simulink model "QuadcopterModel"  (R2021b)
settings: Solver=VariableStepAuto  StartTime=0  StopTime=20  RelTol=1e-3
values from neighbouring files (symbols this model uses):
  b = 3.59 * 10^(-5)    (= 3.59e-05)    [LQR_controller.m]
  d = 2.081 * 10^(-6)    (= 2.081e-06)    [LQR_controller.m]
  g = 9.81    [LQR_controller.m]
  Ix = 0.00963    [LQR_controller.m]
  Iy = 0.00963    [LQR_controller.m]
  Iz = 0.019    [LQR_controller.m]
  Jr = 5.225 * 10^(-5)    (= 5.225e-05)    [LQR_controller.m]
  l = 0.24    [LQR_controller.m]
  m = 0.9928    [LQR_controller.m]
undefined symbols (not defined in the file or in its folder): rad, s, sigbuilder_block
libraries: slpidlib x7, simulink_extras x2, aerolibconvert2 x1
settings Model: Creator=sevba  LastModifiedBy=SEVBAN ALTAY
settings SolverCC: ZeroCrossAlgorithm=Adaptive
settings DataIOCC: SaveFormat=StructureWithTime
settings OptimizationCC: BlockReduction=off  BufferReuse=off
settings DebuggingCC: AlgebraicLoopMsg=none  IgnoredZcDiagnostic=none  UnconnectedInputMsg=none  UnconnectedOutputMsg=none  UnconnectedLineMsg=none
settings ExplorerConfigSet: SimMechanicsOpenEditorOnUpdate=off

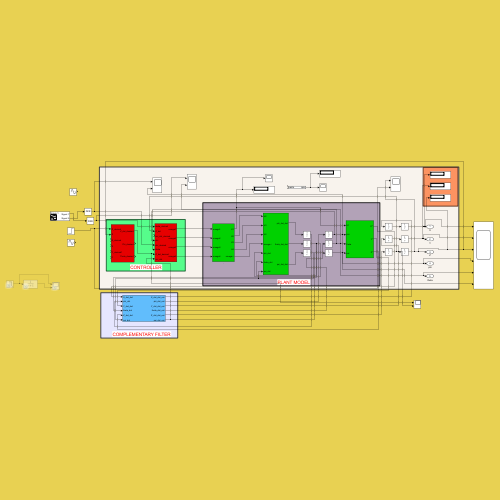
[thumbnail: Simulink's stored preview of the top-level diagram]
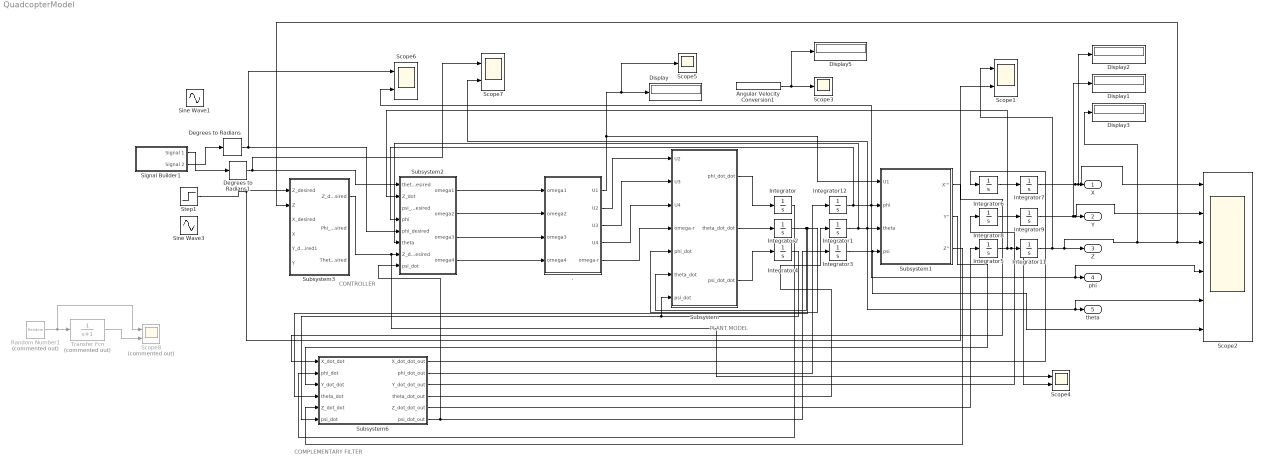
== system QuadcopterModel ==
  note: PLANT MODEL
  note: CONTROLLER
  note: COMPLEMENTARY FILTER
  . : Subsystem
  Angular Velocity Conversion1 : aerolibconvert2/Angular Velocity Conversion  IU=rad/s  OU=rpm
  Degrees to Radians : simulink_extras/Transformations/Degrees to Radians
  Degrees to Radians1 : simulink_extras/Transformations/Degrees to Radians
  Display{,1..3,5} (5 alike) : Display
  Integrator{,1..7,9,12} (10 alike) : Integrator
  Integrator11 : Integrator  UpperSaturationLimit=0  WrappedStateUpperValue=0
  Integrator8 : Integrator  UpperSaturationLimit=0
  Random Number1 : RandomNumber  Commented=on  Variance=0.0001  Seed=1  SampleTime=0.01
  Scope{1,4,6..7} (4 alike) : Scope  NumInputPorts=2
  Scope2 : Scope  NumInputPorts=6
  Scope3 : Scope
  Scope5 : Scope
  Scope8 : Scope  Commented=on  NumInputPorts=2
  Signal Builder1 : Subsystem  Tag=STV Subsys  LoadFcn=sigbuilder_block('load');  StartFcn=sigbuilder_block('start');  StopFcn=sigbuilder_block('stop');  ClipboardFcn=sigbuilder_block('clipboard');  mask(Sigbuilder block){tuvar=[0:10]}
      mask help: Simulink:masks:SigbuilderBlock_MD
      mask init:
      | if ~strcmp(get_param(bdroot(gcbh),'SimulationStatus'),'stopped') tuvar = sigbuilder_block('maskInit'); end
      settings: CopyFcn=sigbuilder_block('copy');  DeleteFcn=sigbuilder_block('delete');  ModelCloseFcn=sigbuilder_block('modelClose');  PreSaveFcn=sigbuilder_block('preSave');  PauseFcn=sigbuilder_block('pause');  ContinueFcn=sigbuilder_block('continue');  NameChangeFcn=sigbuilder_block('namechange');  OpenFcn=sigbuilder_block('open',[182.4 96.6 550.8 400.2 ]);  CloseFcn=sigbuilder_block('close');
      mask Display: plot(0, 0, 100, 100,[2, 2, 32, 32, 2], [68, 8, 8, 68, 68],[32, 2], [38, 38], [32, 19, 2],[53, 60, 44], [32, 17, 17, 2],[16, 16, 31, 31]);txt = getActiveGroup(gcbh);text(2, 100, txt,'verticalAlignment', 'top');
  Sine Wave1 : Sin  SampleTime=0
  Sine Wave3 : Sin  SampleTime=0
  Step1 : Step  SampleTime=0
  Subsystem : Subsystem
  Subsystem1 : Subsystem
  Subsystem2 : Subsystem
  Subsystem3 : Subsystem
  Subsystem6 : Subsystem
  Transfer Fcn : TransferFcn  Commented=on  Denominator=[1 1]
  X : Outport
  "Y " : Outport  Port=2
  Z : Outport  Port=3
  phi : Outport  Port=4
  "theta " : Outport  Port=5
  wires:
  Integrator5/1 -> Scope4/2, Integrator11/1, Subsystem2/2(Z_dot)
  Integrator8/1 -> Integrator9/1
  ./3(U3) -> Subsystem/2(U3)
  ./1(U1) -> Scope5/1, Display/1, Subsystem1/1(U1)
  Integrator3/1 -> Subsystem1/4(psi), Scope2/6
  Subsystem/3(psi_dot_dot) -> Integrator4/1
  Subsystem/2(theta_dot_dot) -> Integrator2/1
  ./2(U2) -> Subsystem/1(U2)
  Integrator2/1 -> Subsystem6/4(theta_dot), Subsystem/5(phi_dot), Subsystem/6(theta_dot)
  Integrator11/1 -> Scope1/1, Subsystem3/2(Z), Scope2/3, Display3/1, Z/1
  Integrator9/1 -> Display1/1, Scope2/2, "Y "/1
  Integrator6/1 -> Integrator7/1
  Integrator12/1 -> Subsystem2/4(phi), phi/1, Scope2/4, Subsystem1/2(phi), Scope6/2
  Subsystem/1(phi_dot_dot) -> Integrator/1
  Integrator4/1 -> Subsystem6/6(psi_dot), Subsystem/7(psi_dot)
  Integrator1/1 -> Subsystem2/6(theta), Scope2/5, "theta "/1, Scope7/2, Subsystem1/3(theta)
  ./4(U4) -> Subsystem/3(U4)
  Angular Velocity Conversion1/1 -> Display5/1, Scope3/1
  Integrator7/1 -> Scope2/1, Display2/1, X/1
  ./5(omega-r) -> Subsystem/4(omega-r)
  Subsystem2/1(omega1) -> ./1(omega1)
  Subsystem2/2(omega2) -> ./2(omega2)
  Subsystem2/3(omega3) -> ./3(omega3)
  Subsystem2/4(omega4) -> ./4(omega4)
  Step1/1 -> Scope1/2, Subsystem3/1(Z_desired)
  Subsystem3/1(Z_dot_desired) -> Scope4/1, Subsystem2/7(Z_dot_desired)
  Degrees to Radians/1 -> Subsystem2/5(phi_desired), Scope6/1
  Subsystem6/6(psi_dot_out) -> Subsystem2/8(psi_dot), Integrator3/1
  Subsystem1/1(X''') -> Subsystem6/1(X_dot_dot)
  Integrator/1 -> Subsystem6/2(phi_dot)
  Subsystem1/2(Y'') -> Subsystem6/3(Y_dot_dot)
  Subsystem6/1(X_dot_dot_out) -> Integrator6/1
  Subsystem6/2(phi_dot_out) -> Integrator12/1
  Subsystem6/3(Y_dot_dot_out) -> Integrator8/1
  Subsystem6/4(theta_dot_out) -> Integrator1/1
  Subsystem6/5(Z_dot_dot_out) -> Integrator5/1
  Subsystem1/3(Z'') -> Subsystem6/5(Z_dot_dot)
  Degrees to Radians1/1 -> Scope7/1, Subsystem2/1(theta_desired)
  Signal Builder1/2(Signal 2) -> Degrees to Radians/1
  Signal Builder1/1(Signal 1) -> Degrees to Radians1/1
  Random Number1/1 -> Scope8/1, Transfer Fcn/1
  Transfer Fcn/1 -> Scope8/2

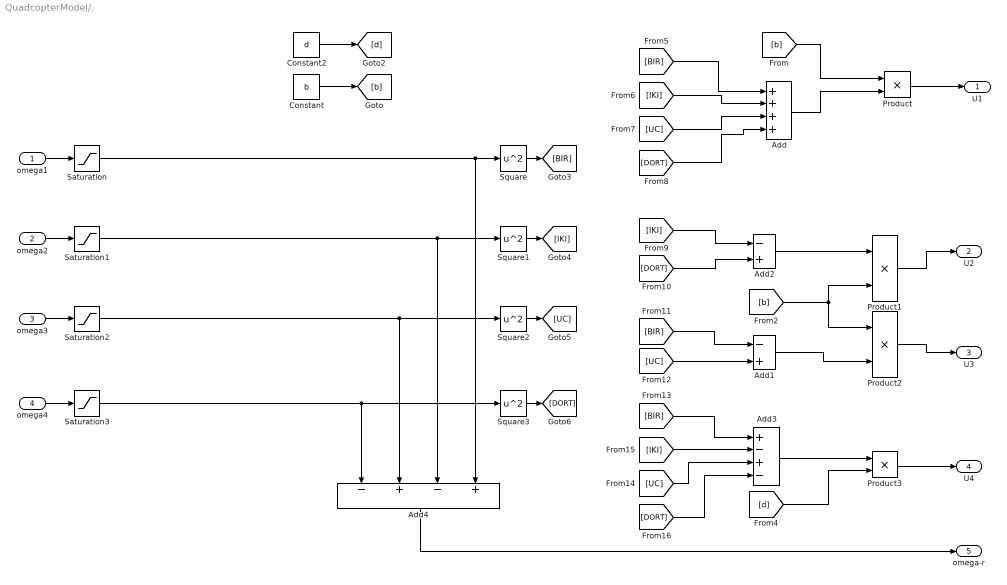
== system QuadcopterModel/. ==
  omega1 : Inport
  omega2 : Inport  Port=2
  omega3 : Inport  Port=3
  omega4 : Inport  Port=4
  Add : Sum  Inputs=++++
  Add1 : Sum  Inputs=-+
  Add2 : Sum  Inputs=-+
  Add3 : Sum  Inputs=+-+-
  Add4 : Sum  Inputs=-+-+
  Constant : Constant  Value=b
  Constant2 : Constant  Value=d
  Product{,1..3} (4 alike) : Product
  Saturation{,1..3} (4 alike) : Saturate  UpperLimit=inf  LowerLimit=0
  Square{,1..3} (4 alike) : Math  Operator=square  SaturateOnIntegerOverflow=on
  U1 : Outport
  U2 : Outport  Port=2
  U3 : Outport  Port=3
  U4 : Outport  Port=4
  omega-r : Outport  Port=5
  wires:
  Add/1 -> Product/2
  Product/1 -> U1/1
  Constant/1 -> [b]
  [b] -> Product/1
  Add2/1 -> Product1/1
  [b] -> Product1/2, Product2/1
  Add1/1 -> Product2/2
  Constant2/1 -> [d]
  Add3/1 -> Product3/1
  [d] -> Product3/2
  Product1/1 -> U2/1
  Product3/1 -> U4/1
  Product2/1 -> U3/1
  Square/1 -> [BIR]
  [BIR] -> Add/1
  Square1/1 -> [IKI]
  [IKI] -> Add/2
  Square2/1 -> [UC]
  [UC] -> Add/3
  Square3/1 -> [DORT]
  [DORT] -> Add/4
  [IKI] -> Add2/1
  [DORT] -> Add2/2
  [BIR] -> Add1/1
  [UC] -> Add1/2
  [BIR] -> Add3/1
  [UC] -> Add3/3
  [IKI] -> Add3/2
  [DORT] -> Add3/4
  Add4/1 -> omega-r/1
  omega1/1 -> Saturation/1
  omega2/1 -> Saturation1/1
  omega3/1 -> Saturation2/1
  omega4/1 -> Saturation3/1
  Saturation/1 -> Add4/4, Square/1
  Saturation1/1 -> Add4/3, Square1/1
  Saturation2/1 -> Add4/2, Square2/1
  Saturation3/1 -> Square3/1, Add4/1

== system QuadcopterModel/Signal Builder1 ==
  Demux : Demux  Tag=STV Demux  Outputs=2
      settings: DisplayOption=none
  FromWs : FromWorkspace  Tag=STV FromWs  VariableName=tuvar
      SigBuilderData=|
      | common.afterFinalStr = 'Extrapolate'
      | common.sampleTime = 0
      | dataSet.timeRange = [0 10]
      | dataSet.name = 'Group 1'
      | sbobj.Groups.Name = 'Group 1'
      | sbobj.Groups.Signals(1).Name = 'Signal 1'
      | sbobj.Groups.Signals(1).XData = [0 4 4 6 6 10]
      | sbobj.Groups.Signals(1).YData = [0 0 2.9 2.9 0 0]
      | sbobj.Groups.Signals(2).Name = 'Signal 2'
      | sbobj.Groups.Signals(2).XData = [0 4 4 6 6 10]
      | sbobj.Groups.Signals(2).YData = [0 0 -2.9 -2.9 0 0]
  Signal 1 : Outport  Tag=STV Outport
  Signal 2 : Outport  Tag=STV Outport  Port=2
  wires:
  FromWs/1 -> Demux/1
  Demux/1 -> Signal 1/1
  Demux/2 -> Signal 2/1

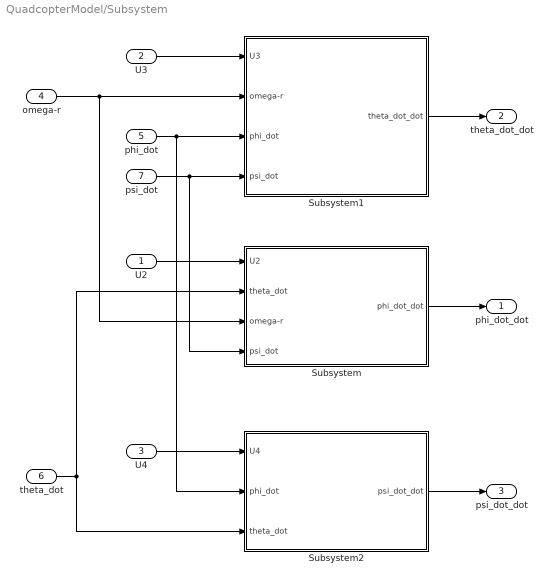
== system QuadcopterModel/Subsystem ==
  U2 : Inport
  U3 : Inport  Port=2
  U4 : Inport  Port=3
  omega-r : Inport  Port=4
  phi_dot : Inport  Port=5
  theta_dot : Inport  Port=6
  psi_dot : Inport  Port=7
  Subsystem : Subsystem
  Subsystem1 : Subsystem
  Subsystem2 : Subsystem
  phi_dot_dot : Outport
  theta_dot_dot : Outport  Port=2
  psi_dot_dot : Outport  Port=3
  wires:
  U2/1 -> Subsystem/1(U2)
  theta_dot/1 -> Subsystem2/3(theta_dot), Subsystem/2(theta_dot)
  psi_dot/1 -> Subsystem/4(psi_dot), Subsystem1/4(psi_dot)
  Subsystem/1(phi_dot_dot) -> phi_dot_dot/1
  U3/1 -> Subsystem1/1(U3)
  Subsystem1/1(theta_dot_dot) -> theta_dot_dot/1
  phi_dot/1 -> Subsystem2/2(phi_dot), Subsystem1/3(phi_dot)
  omega-r/1 -> Subsystem/3(omega-r), Subsystem1/2(omega-r)
  Subsystem2/1(psi_dot_dot) -> psi_dot_dot/1
  U4/1 -> Subsystem2/1(U4)

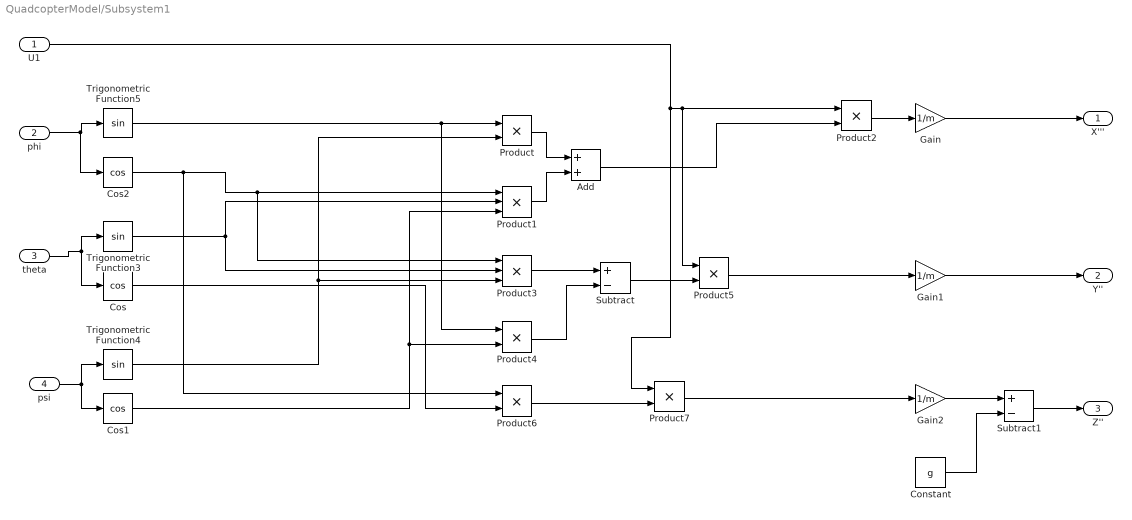
== system QuadcopterModel/Subsystem1 ==
  U1 : Inport
  phi : Inport  Port=2
  theta : Inport  Port=3
  psi : Inport  Port=4
  Add : Sum
  Constant : Constant  Value=g
  Cos : Trigonometry  Operator=cos
  Cos1 : Trigonometry  Operator=cos
  Cos2 : Trigonometry  Operator=cos
  Gain : Gain  Gain=1/m
  Gain1 : Gain  Gain=1/m
  Gain2 : Gain  Gain=1/m
  Product{,2,4..7} (6 alike) : Product
  Product1 : Product  Inputs=3
  Product3 : Product  Inputs=3
  Subtract : Sum  Inputs=+-
  Subtract1 : Sum  Inputs=+-
  Trigonometric Function3 : Trigonometry
  Trigonometric Function4 : Trigonometry
  Trigonometric Function5 : Trigonometry
  X''' : Outport
  Y'' : Outport  Port=2
  Z'' : Outport  Port=3
  wires:
  Constant/1 -> Subtract1/2
  Product5/1 -> Gain1/1
  U1/1 -> Product7/1, Product5/1, Product2/1
  theta/1 -> Trigonometric Function3/1, Cos/1
  phi/1 -> Cos2/1, Trigonometric Function5/1
  Gain2/1 -> Subtract1/1
  Cos1/1 -> Product4/2, Product1/3
  Product3/1 -> Subtract/1
  Cos/1 -> Product6/2
  Product1/1 -> Add/2
  Product2/1 -> Gain/1
  Trigonometric Function3/1 -> Product3/2, Product1/2
  Product4/1 -> Subtract/2
  Add/1 -> Product2/2
  Subtract/1 -> Product5/2
  Trigonometric Function5/1 -> Product4/1, Product/1
  Gain1/1 -> Y''/1
  psi/1 -> Trigonometric Function4/1, Cos1/1
  Gain/1 -> X'''/1
  Subtract1/1 -> Z''/1
  Product/1 -> Add/1
  Trigonometric Function4/1 -> Product3/3, Product/2
  Product7/1 -> Gain2/1
  Product6/1 -> Product7/2
  Cos2/1 -> Product6/1, Product1/1, Product3/1

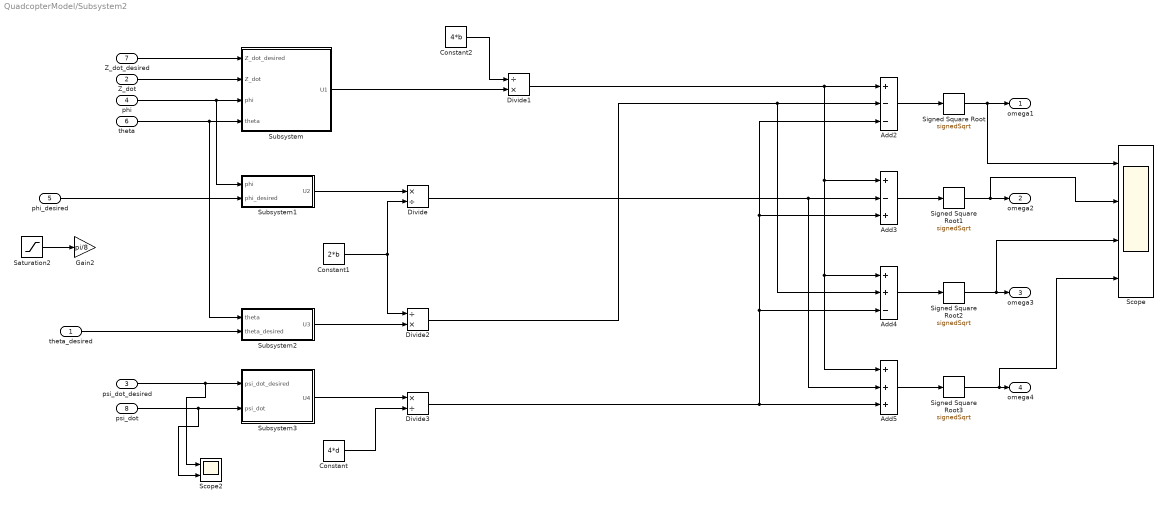
== system QuadcopterModel/Subsystem2 ==
  theta_desired : Inport
  Z_dot : Inport  Port=2
  psi_dot_desired : Inport  Port=3
  phi : Inport  Port=4
  phi_desired : Inport  Port=5
  theta : Inport  Port=6
  Z_dot_desired : Inport  Port=7
  psi_dot : Inport  Port=8
  Add2 : Sum  Inputs=+--
  Add3 : Sum  Inputs=+-+
  Add4 : Sum  Inputs=++-
  Add5 : Sum  Inputs=+++
  Constant : Constant  Value=4*d
  Constant1 : Constant  Value=2*b
  Constant2 : Constant  Value=4*b
  Divide : Product  Inputs=*/
  Divide1 : Product  Inputs=/*
  Divide2 : Product  Inputs=/*
  Divide3 : Product  Inputs=*/
  Gain2 : Gain  Gain=pi/8
  Saturation2 : Saturate  UpperLimit=1  LowerLimit=-1
  Scope : Scope  NumInputPorts=4
  Scope2 : Scope  NumInputPorts=2
  Signed Square Root{,1..3} (4 alike) : Sqrt  Operator=signedSqrt  SaturateOnIntegerOverflow=on
  Subsystem : Subsystem
  Subsystem1 : Subsystem
  Subsystem2 : Subsystem
  Subsystem3 : Subsystem
  omega1 : Outport
  omega2 : Outport  Port=2
  omega3 : Outport  Port=3
  omega4 : Outport  Port=4
  wires:
  theta_desired/1 -> Subsystem2/2(theta_desired)
  Divide1/1 -> Add5/1, Add4/1, Add3/1, Add2/1
  Z_dot/1 -> Subsystem/2(Z_dot)
  Signed Square Root3/1 -> Scope/4, omega4/1
  Constant1/1 -> Divide/2, Divide2/1
  Subsystem2/1(U3) -> Divide2/2
  Add2/1 -> Signed Square Root/1
  Divide/1 -> Add5/2, Add3/2
  Signed Square Root2/1 -> Scope/3, omega3/1
  phi_desired/1 -> Subsystem1/2(phi_desired)
  Signed Square Root/1 -> Scope/1, omega1/1
  Subsystem1/1(U2) -> Divide/1
  Z_dot_desired/1 -> Subsystem/1(Z_dot_desired)
  Signed Square Root1/1 -> Scope/2, omega2/1
  theta/1 -> Subsystem2/1(theta), Subsystem/4(theta)
  psi_dot/1 -> Scope2/2, Subsystem3/2(psi_dot)
  psi_dot_desired/1 -> Scope2/1, Subsystem3/1(psi_dot_desired)
  Constant/1 -> Divide3/2
  Add4/1 -> Signed Square Root2/1
  Subsystem/1(U1) -> Divide1/2
  Add5/1 -> Signed Square Root3/1
  Add3/1 -> Signed Square Root1/1
  Divide3/1 -> Add4/3, Add2/3, Add3/3, Add5/3
  Subsystem3/1(U4) -> Divide3/1
  Divide2/1 -> Add4/2, Add2/2
  Constant2/1 -> Divide1/1
  phi/1 -> Subsystem1/1(phi), Subsystem/3(phi)
  Saturation2/1 -> Gain2/1

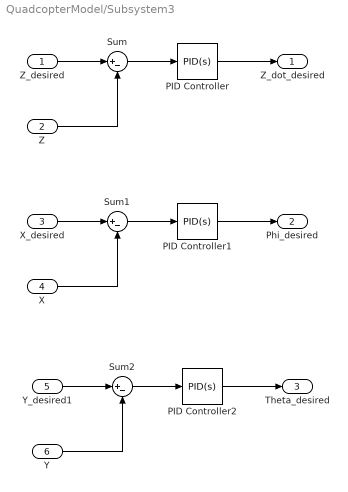
== system QuadcopterModel/Subsystem3 ==
  Z_desired : Inport
  Z : Inport  Port=2
  X_desired : Inport  Port=3
  X : Inport  Port=4
  Y_desired1 : Inport  Port=5
  Y : Inport  Port=6
  PID Controller : slpidlib/PID Controller  Controller=PID  Form=Parallel  TimeDomain=Continuous-time  UseExternalTs=off  SampleTime=-1  IntegratorMethod=Forward Euler  FilterMethod=Forward Euler  ControllerParametersSource=internal  P=10  I=20  D=1  UseFilter=on  N=38.6726288731783  TunerSelectOption=Transfer Function Based (PID Tuner App)  InitialConditionSource=internal  InitialConditionForIntegrator=0  InitialConditionForFilter=0  DifferentiatorICPrevScaledInput=0  ExternalReset=none  TrackingMode=off  Kt=1  LimitOutput=on  SatLimitsSource=internal  UpperSaturationLimit=5  LowerSaturationLimit=-5  LinearizeAsGain=on  AntiWindupMode=clamping  Kb=1  POutMin=[]  POutMax=[]  IOutMin=[]  IOutMax=[]  DOutMin=[]  DOutMax=[]  NOutMin=[]  NOutMax=[]  SumOutMin=[]  SumOutMax=[]  SaturationOutMin=[]  SaturationOutMax=[]  PParamMin=[]  PParamMax=[]  IParamMin=[]  IParamMax=[]  DParamMin=[]  DParamMax=[]  NParamMin=[]  NParamMax=[]  KbParamMin=[]  KbParamMax=[]  KtParamMin=[]  KtParamMax=[]  KbOutMin=[]  KbOutMax=[]  KtOutMin=[]  KtOutMax=[]  IntegratorOutMin=[]  IntegratorOutMax=[]  FilterOutMin=[]  FilterOutMax=[]  SumI1OutMin=[]  SumI1OutMax=[]  SumI2OutMin=[]  SumI2OutMax=[]  SumI3OutMin=[]  SumI3OutMax=[]  SumI4OutMin=[]  SumI4OutMax=[]  SumDOutMin=[]  SumDOutMax=[]  DifferentiatorOutMin=[]  DifferentiatorOutMax=[]  FilterDiffOutCoefMin=[]  FilterDiffOutCoefMax=[]  ReciprocalOutMin=[]  ReciprocalOutMax=[]  SumDenOutMin=[]  SumDenOutMax=[]  SumNumOutMin=[]  SumNumOutMax=[]  DivideOutMin=[]  DivideOutMax=[]  UdiffTsProdOutMin=[]  UdiffTsProdOutMax=[]  NTsProdOutMin=[]  NTsProdOutMax=[]  UintegralTsProdOutMin=[]  UintegralTsProdOutMax=[]  UngainTsProdOutMin=[]  UngainTsProdOutMax=[]  IntegratorContinuousStateAttributes=''  IntegratorStateMustResolveToSignalObject=off  IntegratorRTWStateStorageClass=Auto  FilterContinuousStateAttributes=''  FilterStateMustResolveToSignalObject=off  FilterRTWStateStorageClass=Auto  ParallelPVariant=InternalParameters  IdealPVariant=Disabled  IVariant=InternalParameters  DVariant=InternalParameters  IntegratorVariant=Continuous  SatVariant=Enabled  AWVariant=ContClampingParallel  PCopyVariant=Disabled  TRVariant=Disabled  FdbkBlocksVariant=Forward  IdealPFdbkVariant=Disabled  SatFdbkVariant=Disabled  DerivativeFilterVariant=ContFilter  NVariant=InternalParameters  NCopyVariant=Disabled  FilterICVariant=InternalICsFilter  IntegratorICVariant=InternalICs  ExternalResetVariant=Disabled  TRSumVariant=Passthrough  SumFdbkVariant=Disabled  SumVariant=Sum_PID  TsampFilterVariant=InternalTs  TsampNgainVariant=Passthrough  TsampIntegralVariant=Passthrough  ExternalSaturationOutDataTypeStr=Inherit: Same as second input
  PID Controller1 : slpidlib/PID Controller  Controller=PID  Form=Parallel  TimeDomain=Continuous-time  UseExternalTs=off  SampleTime=-1  IntegratorMethod=Forward Euler  FilterMethod=Forward Euler  ControllerParametersSource=internal  P=-0.717  I=-0.287  D=-1.11  UseFilter=on  N=50  TunerSelectOption=Transfer Function Based (PID Tuner App)  InitialConditionSource=internal  InitialConditionForIntegrator=0  InitialConditionForFilter=0  DifferentiatorICPrevScaledInput=0  ExternalReset=none  TrackingMode=off  Kt=1  LimitOutput=on  SatLimitsSource=internal  UpperSaturationLimit=5  LowerSaturationLimit=-5  LinearizeAsGain=on  AntiWindupMode=clamping  Kb=1  POutMin=[]  POutMax=[]  IOutMin=[]  IOutMax=[]  DOutMin=[]  DOutMax=[]  NOutMin=[]  NOutMax=[]  SumOutMin=[]  SumOutMax=[]  SaturationOutMin=[]  SaturationOutMax=[]  PParamMin=[]  PParamMax=[]  IParamMin=[]  IParamMax=[]  DParamMin=[]  DParamMax=[]  NParamMin=[]  NParamMax=[]  KbParamMin=[]  KbParamMax=[]  KtParamMin=[]  KtParamMax=[]  KbOutMin=[]  KbOutMax=[]  KtOutMin=[]  KtOutMax=[]  IntegratorOutMin=[]  IntegratorOutMax=[]  FilterOutMin=[]  FilterOutMax=[]  SumI1OutMin=[]  SumI1OutMax=[]  SumI2OutMin=[]  SumI2OutMax=[]  SumI3OutMin=[]  SumI3OutMax=[]  SumI4OutMin=[]  SumI4OutMax=[]  SumDOutMin=[]  SumDOutMax=[]  DifferentiatorOutMin=[]  DifferentiatorOutMax=[]  FilterDiffOutCoefMin=[]  FilterDiffOutCoefMax=[]  ReciprocalOutMin=[]  ReciprocalOutMax=[]  SumDenOutMin=[]  SumDenOutMax=[]  SumNumOutMin=[]  SumNumOutMax=[]  DivideOutMin=[]  DivideOutMax=[]  UdiffTsProdOutMin=[]  UdiffTsProdOutMax=[]  NTsProdOutMin=[]  NTsProdOutMax=[]  UintegralTsProdOutMin=[]  UintegralTsProdOutMax=[]  UngainTsProdOutMin=[]  UngainTsProdOutMax=[]  IntegratorContinuousStateAttributes=''  IntegratorStateMustResolveToSignalObject=off  IntegratorRTWStateStorageClass=Auto  FilterContinuousStateAttributes=''  FilterStateMustResolveToSignalObject=off  FilterRTWStateStorageClass=Auto  ParallelPVariant=InternalParameters  IdealPVariant=Disabled  IVariant=InternalParameters  DVariant=InternalParameters  IntegratorVariant=Continuous  SatVariant=Enabled  AWVariant=ContClampingParallel  PCopyVariant=Disabled  TRVariant=Disabled  FdbkBlocksVariant=Forward  IdealPFdbkVariant=Disabled  SatFdbkVariant=Disabled  DerivativeFilterVariant=ContFilter  NVariant=InternalParameters  NCopyVariant=Disabled  FilterICVariant=InternalICsFilter  IntegratorICVariant=InternalICs  ExternalResetVariant=Disabled  TRSumVariant=Passthrough  SumFdbkVariant=Disabled  SumVariant=Sum_PID  TsampFilterVariant=InternalTs  TsampNgainVariant=Passthrough  TsampIntegralVariant=Passthrough  ExternalSaturationOutDataTypeStr=Inherit: Same as second input
  PID Controller2 : slpidlib/PID Controller  Controller=PID  Form=Parallel  TimeDomain=Continuous-time  UseExternalTs=off  SampleTime=-1  IntegratorMethod=Forward Euler  FilterMethod=Forward Euler  ControllerParametersSource=internal  P=7  I=1.02  D=5.06  UseFilter=on  N=50  TunerSelectOption=Transfer Function Based (PID Tuner App)  InitialConditionSource=internal  InitialConditionForIntegrator=0  InitialConditionForFilter=0  DifferentiatorICPrevScaledInput=0  ExternalReset=none  TrackingMode=off  Kt=1  LimitOutput=off  SatLimitsSource=internal  UpperSaturationLimit=5  LowerSaturationLimit=-5  LinearizeAsGain=on  AntiWindupMode=clamping  Kb=1  POutMin=[]  POutMax=[]  IOutMin=[]  IOutMax=[]  DOutMin=[]  DOutMax=[]  NOutMin=[]  NOutMax=[]  SumOutMin=[]  SumOutMax=[]  SaturationOutMin=[]  SaturationOutMax=[]  PParamMin=[]  PParamMax=[]  IParamMin=[]  IParamMax=[]  DParamMin=[]  DParamMax=[]  NParamMin=[]  NParamMax=[]  KbParamMin=[]  KbParamMax=[]  KtParamMin=[]  KtParamMax=[]  KbOutMin=[]  KbOutMax=[]  KtOutMin=[]  KtOutMax=[]  IntegratorOutMin=[]  IntegratorOutMax=[]  FilterOutMin=[]  FilterOutMax=[]  SumI1OutMin=[]  SumI1OutMax=[]  SumI2OutMin=[]  SumI2OutMax=[]  SumI3OutMin=[]  SumI3OutMax=[]  SumI4OutMin=[]  SumI4OutMax=[]  SumDOutMin=[]  SumDOutMax=[]  DifferentiatorOutMin=[]  DifferentiatorOutMax=[]  FilterDiffOutCoefMin=[]  FilterDiffOutCoefMax=[]  ReciprocalOutMin=[]  ReciprocalOutMax=[]  SumDenOutMin=[]  SumDenOutMax=[]  SumNumOutMin=[]  SumNumOutMax=[]  DivideOutMin=[]  DivideOutMax=[]  UdiffTsProdOutMin=[]  UdiffTsProdOutMax=[]  NTsProdOutMin=[]  NTsProdOutMax=[]  UintegralTsProdOutMin=[]  UintegralTsProdOutMax=[]  UngainTsProdOutMin=[]  UngainTsProdOutMax=[]  IntegratorContinuousStateAttributes=''  IntegratorStateMustResolveToSignalObject=off  IntegratorRTWStateStorageClass=Auto  FilterContinuousStateAttributes=''  FilterStateMustResolveToSignalObject=off  FilterRTWStateStorageClass=Auto  ParallelPVariant=InternalParameters  IdealPVariant=Disabled  IVariant=InternalParameters  DVariant=InternalParameters  IntegratorVariant=Continuous  SatVariant=Disabled  AWVariant=Passthrough  PCopyVariant=Disabled  TRVariant=Disabled  FdbkBlocksVariant=Forward  IdealPFdbkVariant=Disabled  SatFdbkVariant=Disabled  DerivativeFilterVariant=ContFilter  NVariant=InternalParameters  NCopyVariant=Disabled  FilterICVariant=InternalICsFilter  IntegratorICVariant=InternalICs  ExternalResetVariant=Disabled  TRSumVariant=Passthrough  SumFdbkVariant=Disabled  SumVariant=Sum_PID  TsampFilterVariant=InternalTs  TsampNgainVariant=Passthrough  TsampIntegralVariant=Passthrough  ExternalSaturationOutDataTypeStr=Inherit: Same as second input
  Sum : Sum  Inputs=|+-
  Sum1 : Sum  Inputs=|+-
  Sum2 : Sum  Inputs=|+-
  Z_dot_desired : Outport
  Phi_desired : Outport  Port=2
  Theta_desired : Outport  Port=3
  wires:
  Z/1 -> Sum/2
  Z_desired/1 -> Sum/1
  Sum/1 -> PID Controller/1
  PID Controller/1 -> Z_dot_desired/1
  X_desired/1 -> Sum1/1
  PID Controller1/1 -> Phi_desired/1
  X/1 -> Sum1/2
  Sum1/1 -> PID Controller1/1
  Y/1 -> Sum2/2
  PID Controller2/1 -> Theta_desired/1
  Y_desired1/1 -> Sum2/1
  Sum2/1 -> PID Controller2/1

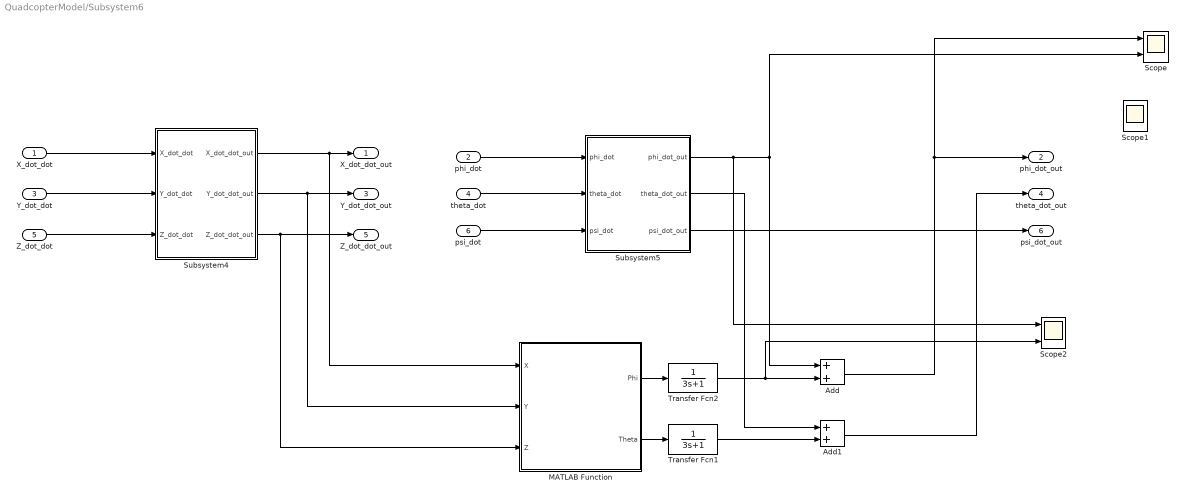
== system QuadcopterModel/Subsystem6 ==
  X_dot_dot : Inport
  phi_dot : Inport  Port=2
  Y_dot_dot : Inport  Port=3
  theta_dot : Inport  Port=4
  Z_dot_dot : Inport  Port=5
  psi_dot : Inport  Port=6
  Add : Sum
  Add1 : Sum
  MATLAB Function : MATLAB Function  TreatAsAtomicUnit=on
  Scope : Scope  NumInputPorts=2
  Scope1 : Scope  NumInputPorts=2
  Scope2 : Scope  NumInputPorts=2
  Subsystem4 : Subsystem
  Subsystem5 : Subsystem
  Transfer Fcn1 : TransferFcn  Denominator=[3 1]
  Transfer Fcn2 : TransferFcn  Denominator=[3 1]
  X_dot_dot_out : Outport
  phi_dot_out : Outport  Port=2
  Y_dot_dot_out : Outport  Port=3
  theta_dot_out : Outport  Port=4
  Z_dot_dot_out : Outport  Port=5
  psi_dot_out : Outport  Port=6
  wires:
  psi_dot/1 -> Subsystem5/3(psi_dot)
  theta_dot/1 -> Subsystem5/2(theta_dot)
  Subsystem4/2(Y_dot_dot_out) -> MATLAB Function/2(Y), Y_dot_dot_out/1
  phi_dot/1 -> Subsystem5/1(phi_dot)
  Subsystem4/1(X_dot_dot_out) -> MATLAB Function/1(X), X_dot_dot_out/1
  Subsystem4/3(Z_dot_dot_out) -> MATLAB Function/3(Z), Z_dot_dot_out/1
  Subsystem5/3(psi_dot_out) -> psi_dot_out/1
  Y_dot_dot/1 -> Subsystem4/2(Y_dot_dot)
  Z_dot_dot/1 -> Subsystem4/3(Z_dot_dot)
  X_dot_dot/1 -> Subsystem4/1(X_dot_dot)
  MATLAB Function/1(Phi) -> Transfer Fcn2/1
  MATLAB Function/2(Theta) -> Transfer Fcn1/1
  Transfer Fcn2/1 -> Scope2/2, Add/2
  Transfer Fcn1/1 -> Add1/2
  Subsystem5/1(phi_dot_out) -> Scope2/1, Scope/2, Add/1
  Subsystem5/2(theta_dot_out) -> Add1/1
  Add/1 -> phi_dot_out/1, Scope/1
  Add1/1 -> theta_dot_out/1

== system QuadcopterModel/Subsystem/Subsystem ==
  U2 : Inport
  theta_dot : Inport  Port=2
  omega-r : Inport  Port=3
  psi_dot : Inport  Port=4
  Add1 : Sum  Inputs=+++
  Gain3 : Gain  Gain=1/Ix
  Jr1 : Constant  Value=Jr
  Product3 : Product
  Product4 : Product  Inputs=3
  Product5 : Product  Inputs=3
  l2 : Constant  Value=l
  l3 : Constant  Value=Iy - Iz
  phi_dot_dot : Outport
  wires:
  Jr1/1 -> Product4/1
  theta_dot/1 -> Product5/1, Product4/2
  psi_dot/1 -> Product5/2
  omega-r/1 -> Product4/3
  l2/1 -> Product3/1
  Product4/1 -> Add1/2
  Add1/1 -> Gain3/1
  l3/1 -> Product5/3
  Product3/1 -> Add1/1
  Product5/1 -> Add1/3
  U2/1 -> Product3/2
  Gain3/1 -> phi_dot_dot/1

== system QuadcopterModel/Subsystem/Subsystem1 ==
  U3 : Inport
  omega-r : Inport  Port=2
  phi_dot : Inport  Port=3
  psi_dot : Inport  Port=4
  Add2 : Sum  Inputs=+++
  Gain1 : Gain  Gain=1/Iy
  Iz-Ix : Constant  Value=Iz - Ix
  Jr : Constant  Value=Jr
  Product1 : Product
  Product2 : Product  Inputs=3
  Product6 : Product  Inputs=3
  l : Constant  Value=l
  theta_dot_dot : Outport
  wires:
  l/1 -> Product1/1
  phi_dot/1 -> Product6/1, Product2/3
  omega-r/1 -> Product2/2
  Jr/1 -> Product2/1
  Iz-Ix/1 -> Product6/3
  psi_dot/1 -> Product6/2
  Product1/1 -> Add2/1
  U3/1 -> Product1/2
  Product2/1 -> Add2/2
  Gain1/1 -> theta_dot_dot/1
  Product6/1 -> Add2/3
  Add2/1 -> Gain1/1

== system QuadcopterModel/Subsystem/Subsystem2 ==
  U4 : Inport
  phi_dot : Inport  Port=2
  theta_dot : Inport  Port=3
  Add1 : Sum
  Gain3 : Gain  Gain=1/Iz
  Product5 : Product  Inputs=3
  lx-Iy : Constant  Value=Ix - Iy
  psi_dot_dot : Outport
  wires:
  phi_dot/1 -> Product5/2
  Add1/1 -> Gain3/1
  lx-Iy/1 -> Product5/3
  U4/1 -> Add1/1
  Product5/1 -> Add1/2
  Gain3/1 -> psi_dot_dot/1
  theta_dot/1 -> Product5/1

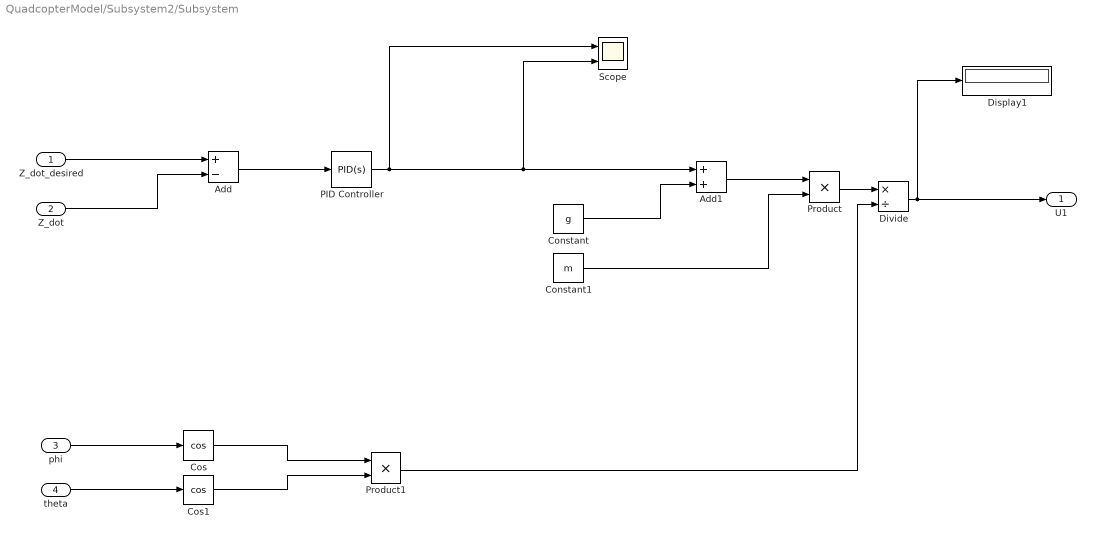
== system QuadcopterModel/Subsystem2/Subsystem ==
  Z_dot_desired : Inport
  Z_dot : Inport  Port=2
  phi : Inport  Port=3
  theta : Inport  Port=4
  Add : Sum  Inputs=+-
  Add1 : Sum
  Constant : Constant  Value=g
  Constant1 : Constant  Value=m
  Cos : Trigonometry  Operator=cos
  Cos1 : Trigonometry  Operator=cos
  Display1 : Display
  Divide : Product  Inputs=*/
  PID Controller : slpidlib/PID Controller  Controller=PID  Form=Parallel  TimeDomain=Continuous-time  UseExternalTs=off  SampleTime=-1  IntegratorMethod=Forward Euler  FilterMethod=Forward Euler  ControllerParametersSource=internal  P=9.53803500543646  I=16.8470505934473  D=0.181138103435098  UseFilter=on  N=36.46824066771  TunerSelectOption=Transfer Function Based (PID Tuner App)  InitialConditionSource=internal  InitialConditionForIntegrator=0  InitialConditionForFilter=0  DifferentiatorICPrevScaledInput=0  ExternalReset=none  TrackingMode=off  Kt=1  LimitOutput=on  SatLimitsSource=internal  UpperSaturationLimit=20  LowerSaturationLimit=-10  LinearizeAsGain=on  AntiWindupMode=back-calculation  Kb=1  POutMin=[]  POutMax=[]  IOutMin=[]  IOutMax=[]  DOutMin=[]  DOutMax=[]  NOutMin=[]  NOutMax=[]  SumOutMin=[]  SumOutMax=[]  SaturationOutMin=[]  SaturationOutMax=[]  PParamMin=[]  PParamMax=[]  IParamMin=[]  IParamMax=[]  DParamMin=[]  DParamMax=[]  NParamMin=[]  NParamMax=[]  KbParamMin=[]  KbParamMax=[]  KtParamMin=[]  KtParamMax=[]  KbOutMin=[]  KbOutMax=[]  KtOutMin=[]  KtOutMax=[]  IntegratorOutMin=[]  IntegratorOutMax=[]  FilterOutMin=[]  FilterOutMax=[]  SumI1OutMin=[]  SumI1OutMax=[]  SumI2OutMin=[]  SumI2OutMax=[]  SumI3OutMin=[]  SumI3OutMax=[]  SumI4OutMin=[]  SumI4OutMax=[]  SumDOutMin=[]  SumDOutMax=[]  DifferentiatorOutMin=[]  DifferentiatorOutMax=[]  FilterDiffOutCoefMin=[]  FilterDiffOutCoefMax=[]  ReciprocalOutMin=[]  ReciprocalOutMax=[]  SumDenOutMin=[]  SumDenOutMax=[]  SumNumOutMin=[]  SumNumOutMax=[]  DivideOutMin=[]  DivideOutMax=[]  UdiffTsProdOutMin=[]  UdiffTsProdOutMax=[]  NTsProdOutMin=[]  NTsProdOutMax=[]  UintegralTsProdOutMin=[]  UintegralTsProdOutMax=[]  UngainTsProdOutMin=[]  UngainTsProdOutMax=[]  IntegratorContinuousStateAttributes=''  IntegratorStateMustResolveToSignalObject=off  IntegratorRTWStateStorageClass=Auto  FilterContinuousStateAttributes=''  FilterStateMustResolveToSignalObject=off  FilterRTWStateStorageClass=Auto  ParallelPVariant=InternalParameters  IdealPVariant=Disabled  IVariant=InternalParameters  DVariant=InternalParameters  IntegratorVariant=Continuous  SatVariant=Enabled  AWVariant=BackCalculation  PCopyVariant=Disabled  TRVariant=Disabled  FdbkBlocksVariant=Forward  IdealPFdbkVariant=Disabled  SatFdbkVariant=Disabled  DerivativeFilterVariant=ContFilter  NVariant=InternalParameters  NCopyVariant=Disabled  FilterICVariant=InternalICsFilter  IntegratorICVariant=InternalICs  ExternalResetVariant=Disabled  TRSumVariant=Passthrough  SumFdbkVariant=Disabled  SumVariant=Sum_PID  TsampFilterVariant=InternalTs  TsampNgainVariant=Passthrough  TsampIntegralVariant=Passthrough  ExternalSaturationOutDataTypeStr=Inherit: Same as second input
  Product : Product
  Product1 : Product
  Scope : Scope  NumInputPorts=2
  U1 : Outport
  wires:
  Product/1 -> Divide/1
  theta/1 -> Cos1/1
  Cos1/1 -> Product1/2
  Cos/1 -> Product1/1
  Product1/1 -> Divide/2
  Add1/1 -> Product/1
  phi/1 -> Cos/1
  Add/1 -> PID Controller/1
  Divide/1 -> Display1/1, U1/1
  Z_dot_desired/1 -> Add/1
  Constant/1 -> Add1/2
  Constant1/1 -> Product/2
  Z_dot/1 -> Add/2
  PID Controller/1 -> Scope/2, Add1/1, Scope/1

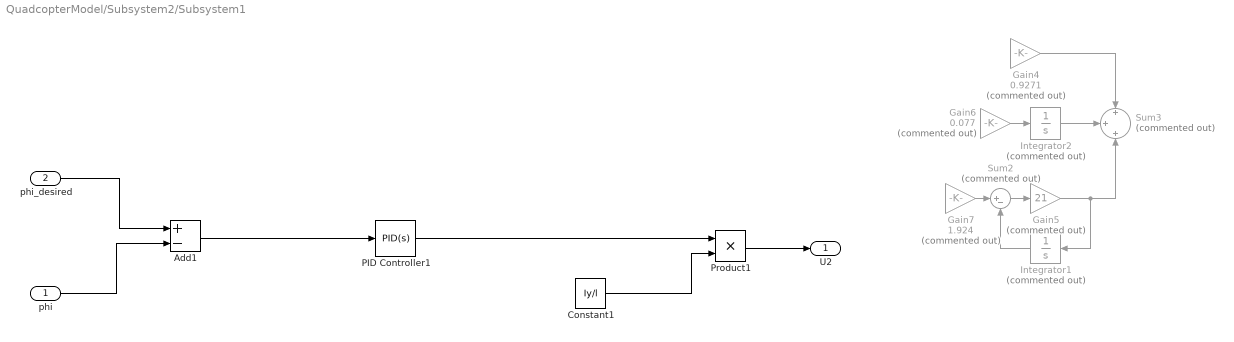
== system QuadcopterModel/Subsystem2/Subsystem1 ==
  phi : Inport
  phi_desired : Inport  Port=2
  Add1 : Sum  Inputs=+-
  Constant1 : Constant  Value=Iy/l
  Gain4 : Gain  Commented=on  Gain=0.9271
  Gain5 : Gain  Commented=on  Gain=21
  Gain6 : Gain  Commented=on  Gain=0.077
  Gain7 : Gain  Commented=on  Gain=1.924
  Integrator1 : Integrator  Commented=on
  Integrator2 : Integrator  Commented=on
  PID Controller1 : slpidlib/PID Controller  Controller=PID  Form=Parallel  TimeDomain=Continuous-time  UseExternalTs=off  SampleTime=-1  IntegratorMethod=Forward Euler  FilterMethod=Forward Euler  ControllerParametersSource=internal  P=96.6269276456994  I=6.81760840912222  D=230.431001888537  UseFilter=on  N=1172.56796225239  TunerSelectOption=Transfer Function Based (PID Tuner App)  InitialConditionSource=internal  InitialConditionForIntegrator=0  InitialConditionForFilter=0  DifferentiatorICPrevScaledInput=0  ExternalReset=none  TrackingMode=off  Kt=1  LimitOutput=off  SatLimitsSource=internal  UpperSaturationLimit=5  LowerSaturationLimit=-5  LinearizeAsGain=on  AntiWindupMode=clamping  Kb=1  POutMin=[]  POutMax=[]  IOutMin=[]  IOutMax=[]  DOutMin=[]  DOutMax=[]  NOutMin=[]  NOutMax=[]  SumOutMin=[]  SumOutMax=[]  SaturationOutMin=[]  SaturationOutMax=[]  PParamMin=[]  PParamMax=[]  IParamMin=[]  IParamMax=[]  DParamMin=[]  DParamMax=[]  NParamMin=[]  NParamMax=[]  KbParamMin=[]  KbParamMax=[]  KtParamMin=[]  KtParamMax=[]  KbOutMin=[]  KbOutMax=[]  KtOutMin=[]  KtOutMax=[]  IntegratorOutMin=[]  IntegratorOutMax=[]  FilterOutMin=[]  FilterOutMax=[]  SumI1OutMin=[]  SumI1OutMax=[]  SumI2OutMin=[]  SumI2OutMax=[]  SumI3OutMin=[]  SumI3OutMax=[]  SumI4OutMin=[]  SumI4OutMax=[]  SumDOutMin=[]  SumDOutMax=[]  DifferentiatorOutMin=[]  DifferentiatorOutMax=[]  FilterDiffOutCoefMin=[]  FilterDiffOutCoefMax=[]  ReciprocalOutMin=[]  ReciprocalOutMax=[]  SumDenOutMin=[]  SumDenOutMax=[]  SumNumOutMin=[]  SumNumOutMax=[]  DivideOutMin=[]  DivideOutMax=[]  UdiffTsProdOutMin=[]  UdiffTsProdOutMax=[]  NTsProdOutMin=[]  NTsProdOutMax=[]  UintegralTsProdOutMin=[]  UintegralTsProdOutMax=[]  UngainTsProdOutMin=[]  UngainTsProdOutMax=[]  IntegratorContinuousStateAttributes=''  IntegratorStateMustResolveToSignalObject=off  IntegratorRTWStateStorageClass=Auto  FilterContinuousStateAttributes=''  FilterStateMustResolveToSignalObject=off  FilterRTWStateStorageClass=Auto  ParallelPVariant=InternalParameters  IdealPVariant=Disabled  IVariant=InternalParameters  DVariant=InternalParameters  IntegratorVariant=Continuous  SatVariant=Disabled  AWVariant=Passthrough  PCopyVariant=Disabled  TRVariant=Disabled  FdbkBlocksVariant=Forward  IdealPFdbkVariant=Disabled  SatFdbkVariant=Disabled  DerivativeFilterVariant=ContFilter  NVariant=InternalParameters  NCopyVariant=Disabled  FilterICVariant=InternalICsFilter  IntegratorICVariant=InternalICs  ExternalResetVariant=Disabled  TRSumVariant=Passthrough  SumFdbkVariant=Disabled  SumVariant=Sum_PID  TsampFilterVariant=InternalTs  TsampNgainVariant=Passthrough  TsampIntegralVariant=Passthrough  ExternalSaturationOutDataTypeStr=Inherit: Same as second input
  Product1 : Product
  Sum2 : Sum  Commented=on  Inputs=|+-
  Sum3 : Sum  Commented=on  Inputs=+|+|+
  U2 : Outport
  wires:
  PID Controller1/1 -> Product1/1
  Constant1/1 -> Product1/2
  phi/1 -> Add1/2
  phi_desired/1 -> Add1/1
  Product1/1 -> U2/1
  Gain7/1 -> Sum2/1
  Gain4/1 -> Sum3/1
  Gain5/1 -> Sum3/3, Integrator1/1
  ? -> Gain6/1
  ? -> Gain4/1
  Integrator1/1 -> Sum2/2
  ? -> Gain7/1
  Sum2/1 -> Gain5/1
  Integrator2/1 -> Sum3/2
  Gain6/1 -> Integrator2/1
  Add1/1 -> PID Controller1/1

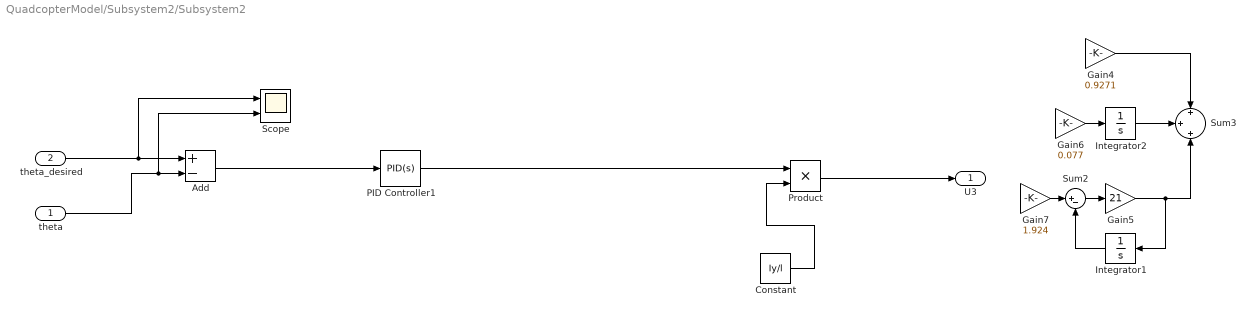
== system QuadcopterModel/Subsystem2/Subsystem2 ==
  theta : Inport
  theta_desired : Inport  Port=2
  Add : Sum  Inputs=+-
  Constant : Constant  Value=Iy/l
  Gain4 : Gain  Gain=0.9271
  Gain5 : Gain  Gain=21
  Gain6 : Gain  Gain=0.077
  Gain7 : Gain  Gain=1.924
  Integrator1 : Integrator
  Integrator2 : Integrator
  PID Controller1 : slpidlib/PID Controller  Controller=PID  Form=Parallel  TimeDomain=Continuous-time  UseExternalTs=off  SampleTime=-1  IntegratorMethod=Forward Euler  FilterMethod=Forward Euler  ControllerParametersSource=internal  P=96.6269276456994  I=6.81760840912222  D=230.431001888537  UseFilter=on  N=1172.56796225239  TunerSelectOption=Transfer Function Based (PID Tuner App)  InitialConditionSource=internal  InitialConditionForIntegrator=0  InitialConditionForFilter=0  DifferentiatorICPrevScaledInput=0  ExternalReset=none  TrackingMode=off  Kt=1  LimitOutput=off  SatLimitsSource=internal  UpperSaturationLimit=5  LowerSaturationLimit=-5  LinearizeAsGain=on  AntiWindupMode=clamping  Kb=1  POutMin=[]  POutMax=[]  IOutMin=[]  IOutMax=[]  DOutMin=[]  DOutMax=[]  NOutMin=[]  NOutMax=[]  SumOutMin=[]  SumOutMax=[]  SaturationOutMin=[]  SaturationOutMax=[]  PParamMin=[]  PParamMax=[]  IParamMin=[]  IParamMax=[]  DParamMin=[]  DParamMax=[]  NParamMin=[]  NParamMax=[]  KbParamMin=[]  KbParamMax=[]  KtParamMin=[]  KtParamMax=[]  KbOutMin=[]  KbOutMax=[]  KtOutMin=[]  KtOutMax=[]  IntegratorOutMin=[]  IntegratorOutMax=[]  FilterOutMin=[]  FilterOutMax=[]  SumI1OutMin=[]  SumI1OutMax=[]  SumI2OutMin=[]  SumI2OutMax=[]  SumI3OutMin=[]  SumI3OutMax=[]  SumI4OutMin=[]  SumI4OutMax=[]  SumDOutMin=[]  SumDOutMax=[]  DifferentiatorOutMin=[]  DifferentiatorOutMax=[]  FilterDiffOutCoefMin=[]  FilterDiffOutCoefMax=[]  ReciprocalOutMin=[]  ReciprocalOutMax=[]  SumDenOutMin=[]  SumDenOutMax=[]  SumNumOutMin=[]  SumNumOutMax=[]  DivideOutMin=[]  DivideOutMax=[]  UdiffTsProdOutMin=[]  UdiffTsProdOutMax=[]  NTsProdOutMin=[]  NTsProdOutMax=[]  UintegralTsProdOutMin=[]  UintegralTsProdOutMax=[]  UngainTsProdOutMin=[]  UngainTsProdOutMax=[]  IntegratorContinuousStateAttributes=''  IntegratorStateMustResolveToSignalObject=off  IntegratorRTWStateStorageClass=Auto  FilterContinuousStateAttributes=''  FilterStateMustResolveToSignalObject=off  FilterRTWStateStorageClass=Auto  ParallelPVariant=InternalParameters  IdealPVariant=Disabled  IVariant=InternalParameters  DVariant=InternalParameters  IntegratorVariant=Continuous  SatVariant=Disabled  AWVariant=Passthrough  PCopyVariant=Disabled  TRVariant=Disabled  FdbkBlocksVariant=Forward  IdealPFdbkVariant=Disabled  SatFdbkVariant=Disabled  DerivativeFilterVariant=ContFilter  NVariant=InternalParameters  NCopyVariant=Disabled  FilterICVariant=InternalICsFilter  IntegratorICVariant=InternalICs  ExternalResetVariant=Disabled  TRSumVariant=Passthrough  SumFdbkVariant=Disabled  SumVariant=Sum_PID  TsampFilterVariant=InternalTs  TsampNgainVariant=Passthrough  TsampIntegralVariant=Passthrough  ExternalSaturationOutDataTypeStr=Inherit: Same as second input
  Product : Product
  Scope : Scope  NumInputPorts=2
  Sum2 : Sum  Inputs=|+-
  Sum3 : Sum  Inputs=+|+|+
  U3 : Outport
  wires:
  theta_desired/1 -> Scope/1, Add/1
  theta/1 -> Scope/2, Add/2
  Constant/1 -> Product/2
  Product/1 -> U3/1
  PID Controller1/1 -> Product/1
  Gain6/1 -> Integrator2/1
  Gain5/1 -> Sum3/3, Integrator1/1
  Integrator2/1 -> Sum3/2
  ? -> Gain7/1, Gain4/1, Gain6/1
  Integrator1/1 -> Sum2/2
  Gain7/1 -> Sum2/1
  Sum2/1 -> Gain5/1
  Gain4/1 -> Sum3/1
  Add/1 -> PID Controller1/1

== system QuadcopterModel/Subsystem2/Subsystem3 ==
  psi_dot_desired : Inport
  psi_dot : Inport  Port=2
  Add : Sum  Inputs=+-
  Constant : Constant  Value=Iz
  PID Controller : slpidlib/PID Controller  Controller=PID  Form=Parallel  TimeDomain=Continuous-time  UseExternalTs=off  SampleTime=-1  IntegratorMethod=Forward Euler  FilterMethod=Forward Euler  ControllerParametersSource=internal  P=-2.92522776752907  I=-1.70549373725632  D=0.265610277194307  UseFilter=on  N=11.0132326144486  TunerSelectOption=Transfer Function Based (PID Tuner App)  InitialConditionSource=internal  InitialConditionForIntegrator=0  InitialConditionForFilter=0  DifferentiatorICPrevScaledInput=0  ExternalReset=none  TrackingMode=off  Kt=1  LimitOutput=off  SatLimitsSource=internal  UpperSaturationLimit=inf  LowerSaturationLimit=-inf  LinearizeAsGain=on  AntiWindupMode=none  Kb=1  POutMin=[]  POutMax=[]  IOutMin=[]  IOutMax=[]  DOutMin=[]  DOutMax=[]  NOutMin=[]  NOutMax=[]  SumOutMin=[]  SumOutMax=[]  SaturationOutMin=[]  SaturationOutMax=[]  PParamMin=[]  PParamMax=[]  IParamMin=[]  IParamMax=[]  DParamMin=[]  DParamMax=[]  NParamMin=[]  NParamMax=[]  KbParamMin=[]  KbParamMax=[]  KtParamMin=[]  KtParamMax=[]  KbOutMin=[]  KbOutMax=[]  KtOutMin=[]  KtOutMax=[]  IntegratorOutMin=[]  IntegratorOutMax=[]  FilterOutMin=[]  FilterOutMax=[]  SumI1OutMin=[]  SumI1OutMax=[]  SumI2OutMin=[]  SumI2OutMax=[]  SumI3OutMin=[]  SumI3OutMax=[]  SumI4OutMin=[]  SumI4OutMax=[]  SumDOutMin=[]  SumDOutMax=[]  DifferentiatorOutMin=[]  DifferentiatorOutMax=[]  FilterDiffOutCoefMin=[]  FilterDiffOutCoefMax=[]  ReciprocalOutMin=[]  ReciprocalOutMax=[]  SumDenOutMin=[]  SumDenOutMax=[]  SumNumOutMin=[]  SumNumOutMax=[]  DivideOutMin=[]  DivideOutMax=[]  UdiffTsProdOutMin=[]  UdiffTsProdOutMax=[]  NTsProdOutMin=[]  NTsProdOutMax=[]  UintegralTsProdOutMin=[]  UintegralTsProdOutMax=[]  UngainTsProdOutMin=[]  UngainTsProdOutMax=[]  IntegratorContinuousStateAttributes=''  IntegratorStateMustResolveToSignalObject=off  IntegratorRTWStateStorageClass=Auto  FilterContinuousStateAttributes=''  FilterStateMustResolveToSignalObject=off  FilterRTWStateStorageClass=Auto  ParallelPVariant=InternalParameters  IdealPVariant=Disabled  IVariant=InternalParameters  DVariant=InternalParameters  IntegratorVariant=Continuous  SatVariant=Disabled  AWVariant=Passthrough  PCopyVariant=Disabled  TRVariant=Disabled  FdbkBlocksVariant=Forward  IdealPFdbkVariant=Disabled  SatFdbkVariant=Disabled  DerivativeFilterVariant=ContFilter  NVariant=InternalParameters  NCopyVariant=Disabled  FilterICVariant=InternalICsFilter  IntegratorICVariant=InternalICs  ExternalResetVariant=Disabled  TRSumVariant=Passthrough  SumFdbkVariant=Disabled  SumVariant=Sum_PID  TsampFilterVariant=InternalTs  TsampNgainVariant=Passthrough  TsampIntegralVariant=Passthrough  ExternalSaturationOutDataTypeStr=Inherit: Same as second input
  Product : Product
  Scope : Scope  NumInputPorts=2
  U4 : Outport
  wires:
  psi_dot_desired/1 -> Scope/1, Add/1
  psi_dot/1 -> Scope/2, Add/2
  Add/1 -> PID Controller/1
  PID Controller/1 -> Product/1
  Constant/1 -> Product/2
  Product/1 -> U4/1

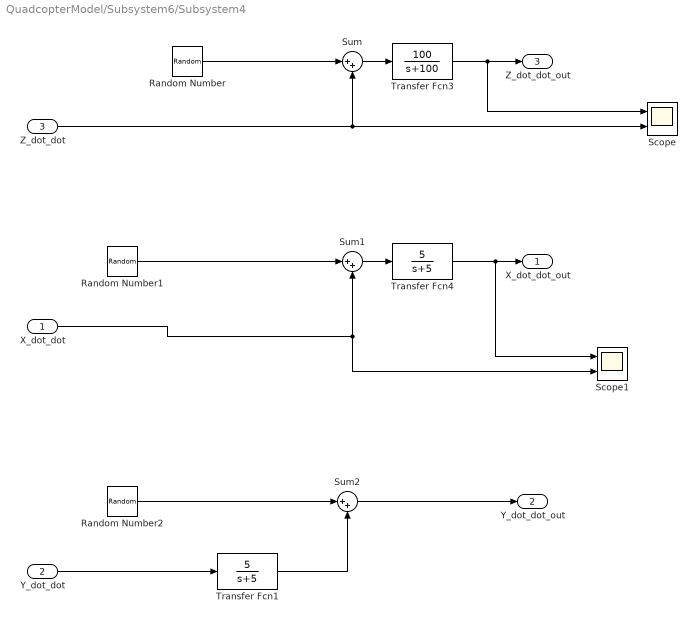
== system QuadcopterModel/Subsystem6/Subsystem4 ==
  X_dot_dot : Inport
  Y_dot_dot : Inport  Port=2
  Z_dot_dot : Inport  Port=3
  Random Number : RandomNumber  Variance=0.001  Seed=1  SampleTime=0.001
  Random Number1 : RandomNumber  Variance=0.0001  Seed=1  SampleTime=0.001
  Random Number2 : RandomNumber  Variance=0.0001  Seed=1  SampleTime=0.001
  Scope : Scope  NumInputPorts=2
  Scope1 : Scope  NumInputPorts=2
  Sum : Sum  Inputs=|++
  Sum1 : Sum  Inputs=|++
  Sum2 : Sum  Inputs=|++
  Transfer Fcn1 : TransferFcn  Numerator=[5]  Denominator=[1 5]
  Transfer Fcn3 : TransferFcn  Numerator=[100]  Denominator=[1 100]
  Transfer Fcn4 : TransferFcn  Numerator=[5]  Denominator=[1 5]
  X_dot_dot_out : Outport
  Y_dot_dot_out : Outport  Port=2
  Z_dot_dot_out : Outport  Port=3
  wires:
  Random Number1/1 -> Sum1/1
  Sum/1 -> Transfer Fcn3/1
  Sum1/1 -> Transfer Fcn4/1
  X_dot_dot/1 -> Sum1/2, Scope1/2
  Y_dot_dot/1 -> Transfer Fcn1/1
  Sum2/1 -> Y_dot_dot_out/1
  Random Number2/1 -> Sum2/1
  Transfer Fcn1/1 -> Sum2/2
  Random Number/1 -> Sum/1
  Transfer Fcn4/1 -> Scope1/1, X_dot_dot_out/1
  Transfer Fcn3/1 -> Scope/1, Z_dot_dot_out/1
  Z_dot_dot/1 -> Scope/2, Sum/2

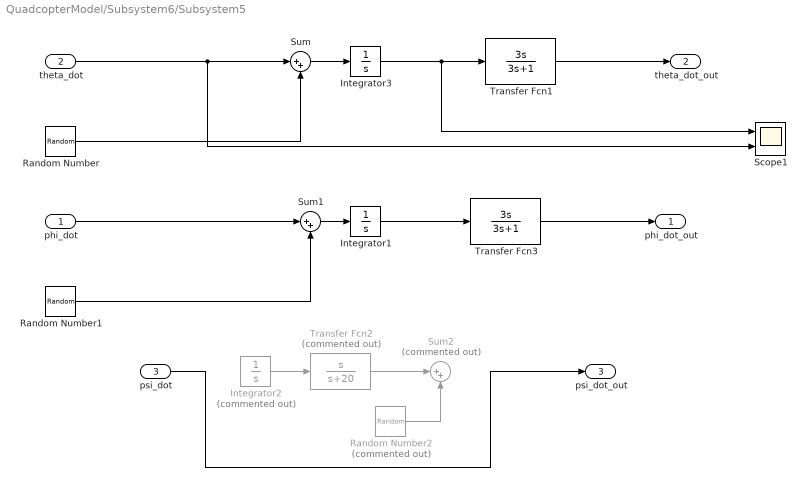
== system QuadcopterModel/Subsystem6/Subsystem5 ==
  phi_dot : Inport
  theta_dot : Inport  Port=2
  psi_dot : Inport  Port=3
  Integrator1 : Integrator
  Integrator2 : Integrator  Commented=on
  Integrator3 : Integrator
  Random Number : RandomNumber  Variance=0.0001  Seed=1  SampleTime=0.001
  Random Number1 : RandomNumber  Variance=0.0001  Seed=1  SampleTime=0.001
  Random Number2 : RandomNumber  Commented=on  Variance=0.0001  Seed=1  SampleTime=0.001
  Scope1 : Scope  NumInputPorts=2
  Sum : Sum  Inputs=|++
  Sum1 : Sum  Inputs=|++
  Sum2 : Sum  Commented=on  Inputs=|++
  Transfer Fcn1 : TransferFcn  Numerator=[3 0]  Denominator=[3 1]
  Transfer Fcn2 : TransferFcn  Commented=on  Numerator=[1 0]  Denominator=[1 20]
  Transfer Fcn3 : TransferFcn  Numerator=[3 0]  Denominator=[3 1]
  phi_dot_out : Outport
  theta_dot_out : Outport  Port=2
  psi_dot_out : Outport  Port=3
  wires:
  phi_dot/1 -> Sum1/1
  Sum1/1 -> Integrator1/1
  theta_dot/1 -> Scope1/2, Sum/1
  Transfer Fcn2/1 -> Sum2/1
  Integrator2/1 -> Transfer Fcn2/1
  Random Number1/1 -> Sum1/2
  Random Number2/1 -> Sum2/2
  psi_dot/1 -> psi_dot_out/1
  Transfer Fcn3/1 -> phi_dot_out/1
  Transfer Fcn1/1 -> theta_dot_out/1
  Random Number/1 -> Sum/2
  Sum/1 -> Integrator3/1
  Integrator3/1 -> Scope1/1, Transfer Fcn1/1
  Integrator1/1 -> Transfer Fcn3/1

== matlab function QuadcopterModel/Subsystem6/MATLAB Function ==
  data: X input; Y input; Phi output; Theta output; Z input
function [Phi, Theta] = Accels2Angles(X,Y,Z)
X_dot_dot=X;
Y_dot_dot=Y;
Z_dot_dot=Z;

Phi=atan(-Y_dot_dot/Z_dot_dot);
Theta=atan(-X_dot_dot/sqrt(Y_dot_dot^2+Z_dot_dot^2));
